simulink model "Example_RPI_Xroad_task"  (Simulink 3.00)
settings: Solver=ode45  SolverMode=SingleTasking  StartTime=0.0  StopTime=10.0  RelTol=1e-3
libraries: logiclib x59, execlib x12, genlib x5, mathlib x4
settings Model: Creator=Jarda  LastModifiedBy=XPMUser

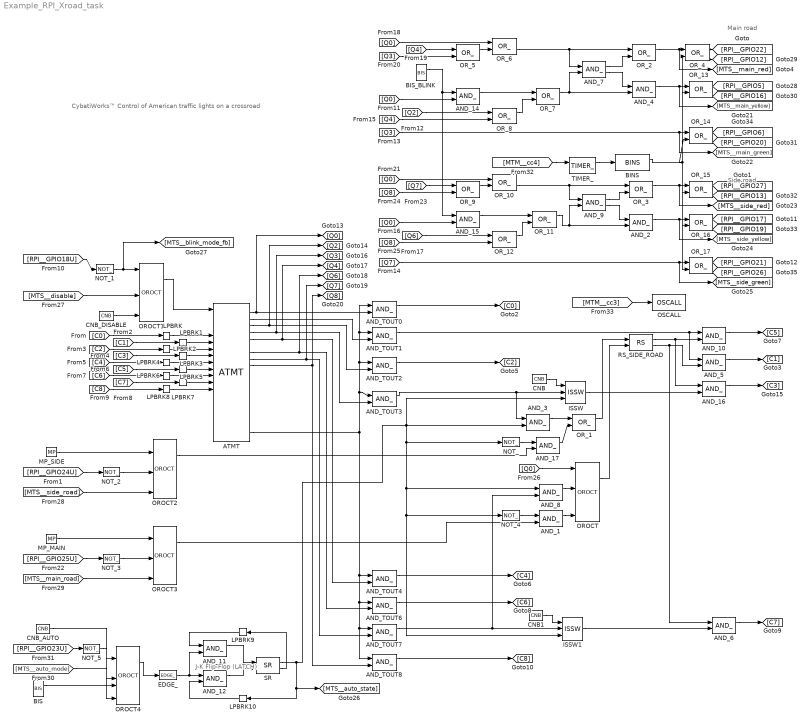
== system Example_RPI_Xroad_task ==
  note: Main road
  note: Side road
  note: J-K Flip-Flop (LATCH)
  note: CybatiWorks™
      | Control of American traffic lights on a crossroad
  AND_{1..12,14..17} (16 alike) : logiclib/AND_
  AND_TOUT{0..4,6..8} (8 alike) : logiclib/AND_
  ATMT : logiclib/ATMT  morestps=off  ntr=9  STT=[0 0 1;1 5 6;1 1 2;2 2 3;3 3 4;4 4 1;6 6 7;7 7 8;8 8 1]  touts=[1 3 2 15 2 0 2 10 2]
  BINS : genlib/BINS  Y0=off  t1=1  t2=2  t3=4  t4=6  t5=8  t6=12  t7=16  t8=20  RPT=off
  BIS : genlib/BIS  Y0=off  t1=1  t2=2  t3=0  t4=0  t5=0  t6=0  t7=0  t8=0  RPT=off
  BIS_BLINK : genlib/BIS  Y0=off  t1=1  t2=2  t3=0  t4=4  t5=5  t6=6  t7=7  t8=8  RPT=on
  CNB : mathlib/CNB  YCN=on
  CNB1 : mathlib/CNB  YCN=on
  CNB_AUTO : mathlib/CNB  YCN=off
  CNB_DISABLE : mathlib/CNB  YCN=off
  EDGE_ : logiclib/EDGE_  iedge=1: Rising edge
  ISSW : logiclib/ISSW
  ISSW1 : logiclib/ISSW
  LPBRK{,1..8} (9 alike) : execlib/LPBRK
  LPBRK10 : execlib/LPBRK  Orientation=left
  LPBRK9 : execlib/LPBRK  Orientation=left
  MP_MAIN : genlib/MP  pwidth=1  BSTATE=off  RPTF=off
  MP_SIDE : genlib/MP  pwidth=1  BSTATE=off  RPTF=off
  NOT_{,1..5} (6 alike) : logiclib/NOT_
  OROCT{,1..4} (5 alike) : logiclib/OROCT  nl=0
  OR_{1..17} (17 alike) : logiclib/OR_
  OSCALL : execlib/OSCALL  action=3: System halt
  RS_SIDE_ROAD : logiclib/RS
  SR : logiclib/SR
  TIMER_ : logiclib/TIMER_  mode=4: Delayed change  pt=1
  wires:
  AND_1/1 -> OROCT/8
  AND_10/1 -> [C5]
  AND_11/1 -> SR/1
  AND_12/1 -> SR/2
  AND_14/1 -> OR_7/1
  AND_15/1 -> OR_11/1
  AND_16/1 -> [C3]
  AND_17/1 -> OR_1/2
  AND_2/1 -> [MTS__side_yellow], OR_16/1
  AND_3/1 -> OR_1/1
  AND_4/1 -> [MTS__main_yellow], OR_13/1
  AND_5/1 -> [C1]
  AND_6/1 -> [C7]
  AND_7/1 -> OR_2/2
  AND_7/2 -> AND_4/1
  AND_8/1 -> OROCT/4
  AND_9/1 -> OR_3/2
  AND_9/2 -> AND_2/1
  AND_TOUT0/1 -> [C0]
  AND_TOUT1/1 -> AND_10/1, AND_5/1
  AND_TOUT2/1 -> [C2]
  AND_TOUT3/1 -> AND_3/1, ISSW/2
  AND_TOUT4/1 -> [C4]
  AND_TOUT6/1 -> [C6]
  AND_TOUT7/1 -> AND_8/2, ISSW1/2
  AND_TOUT8/1 -> [C8]
  ATMT/1 -> AND_TOUT0/2, [Q0]
  ATMT/2 -> AND_TOUT1/2
  ATMT/3 -> AND_TOUT2/2, [Q2]
  ATMT/4 -> AND_TOUT3/2, [Q3]
  ATMT/5 -> AND_TOUT4/2, [Q4]
  ATMT/7 -> AND_TOUT6/2, [Q6]
  ATMT/8 -> AND_TOUT7/2, [Q7]
  ATMT/9 -> AND_TOUT8/2, [Q8]
  ATMT/19 -> AND_TOUT4/1, AND_TOUT6/1, AND_TOUT7/1, AND_TOUT8/1, AND_TOUT3/1, AND_TOUT2/1, AND_TOUT0/1, AND_TOUT1/1
  BINS/1 -> OR_13/2, OR_14/2, OR_15/2, OR_16/2, OR_17/2, OR_4/2
  BIS/1 -> OROCT4/6
  BIS_BLINK/1 -> AND_14/1, AND_15/1
  CNB/1 -> ISSW/1
  CNB1/1 -> ISSW1/1
  CNB_AUTO/1 -> OROCT4/2
  CNB_DISABLE/1 -> OROCT1/8
  EDGE_/1 -> AND_11/2, AND_12/1
  [C0] -> LPBRK/1
  [RPI__GPIO24U] -> NOT_2/1
  [RPI__GPIO18U] -> NOT_1/1
  [Q0] -> AND_14/2
  [Q2] -> OR_8/1
  [Q3] -> [MTS__main_green], OR_14/1
  [Q7] -> [MTS__side_green], OR_17/1
  [Q4] -> OR_8/2
  [Q0] -> AND_15/2
  [Q6] -> OR_12/1
  [Q0] -> OR_6/1
  [Q4] -> OR_5/1
  [C1] -> LPBRK1/1
  [Q3] -> OR_5/2
  [Q0] -> OR_10/1
  [RPI__GPIO25U] -> NOT_3/1
  [Q7] -> OR_9/1
  [Q8] -> OR_9/2
  [Q8] -> OR_12/2
  [Q0] -> OROCT/1
  [MTS__disable] -> OROCT1/5
  [MTS__side_road] -> OROCT2/8
  [MTS__main_road] -> OROCT3/8
  [C2] -> LPBRK2/1
  [MTS__auto_mode] -> OROCT4/8
  [RPI__GPIO23U] -> NOT_5/1
  [MTM__cc4] -> TIMER_/1
  [MTM__cc3] -> OSCALL/1
  [C3] -> LPBRK3/1
  [C4] -> LPBRK4/1
  [C5] -> LPBRK5/1
  [C6] -> LPBRK6/1
  [C7] -> LPBRK7/1
  [C8] -> LPBRK8/1
  ISSW/1 -> AND_16/2
  ISSW1/1 -> AND_6/2
  LPBRK/1 -> ATMT/5
  LPBRK1/1 -> ATMT/6
  LPBRK10/1 -> AND_12/2
  LPBRK2/1 -> ATMT/7
  LPBRK3/1 -> ATMT/8
  LPBRK4/1 -> ATMT/9
  LPBRK5/1 -> ATMT/10
  LPBRK6/1 -> ATMT/11
  LPBRK7/1 -> ATMT/12
  LPBRK8/1 -> ATMT/13
  LPBRK9/1 -> AND_11/1
  MP_MAIN/1 -> OROCT3/2
  MP_SIDE/1 -> OROCT2/2
  NOT_/1 -> AND_17/1
  NOT_1/1 -> [MTS__blink_mode_fb], OROCT1/1
  NOT_2/1 -> OROCT2/5
  NOT_3/1 -> OROCT3/5
  NOT_4/1 -> AND_1/1
  NOT_5/1 -> OROCT4/5
  OROCT/1 -> RS_SIDE_ROAD/2
  OROCT1/1 -> ATMT/1
  OROCT2/1 -> AND_17/2
  OROCT3/1 -> AND_1/2
  OROCT4/1 -> EDGE_/1
  OR_1/1 -> RS_SIDE_ROAD/1
  OR_10/2 -> AND_9/1, OR_3/1
  OR_11/1 -> AND_2/2, AND_9/2
  OR_12/1 -> OR_11/2
  OR_13/1 -> [RPI__GPIO5], [RPI__GPIO16]
  OR_14/1 -> [RPI__GPIO20], [RPI__GPIO6]
  OR_15/1 -> [RPI__GPIO27], [RPI__GPIO13]
  OR_16/1 -> [RPI__GPIO17], [RPI__GPIO19]
  OR_17/1 -> [RPI__GPIO21], [RPI__GPIO26]
  OR_2/1 -> [MTS__main_red], OR_4/1
  OR_3/1 -> [MTS__side_red], OR_15/1
  OR_4/1 -> [RPI__GPIO22], [RPI__GPIO12]
  OR_5/1 -> OR_6/2
  OR_6/2 -> AND_7/1, OR_2/1
  OR_7/1 -> AND_4/2, AND_7/2
  OR_8/1 -> OR_7/2
  OR_9/1 -> OR_10/2
  RS_SIDE_ROAD/1 -> AND_10/2, AND_16/1
  RS_SIDE_ROAD/2 -> AND_5/2, AND_6/1
  SR/1 -> [MTS__auto_state], LPBRK10/1, AND_3/2, NOT_/1, AND_8/1, ISSW1/3, NOT_4/1, ISSW/3
  SR/2 -> LPBRK9/1
  TIMER_/1 -> BINS/1
